simulink model "Bespiel_Architektur_Motor"  (R2025b)
settings: Solver=VariableStepAuto  StartTime=0.0  StopTime=1000  FixedStep=1  RelTol=1e-3
settings Model: DataDictionary=Bespiel_Architektur_Motor_dict.sldd  Creator=P28500  LastModifiedBy=P28500

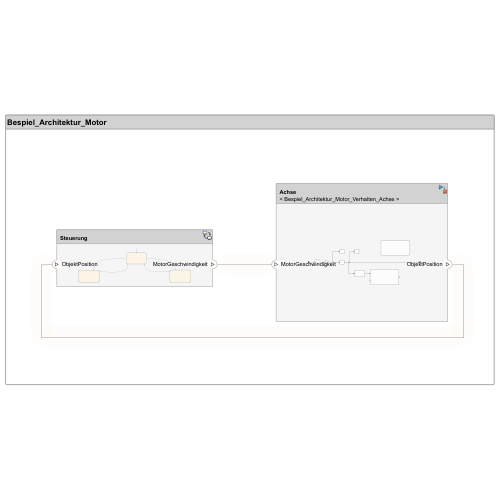
[thumbnail: Simulink's stored preview of the top-level diagram]
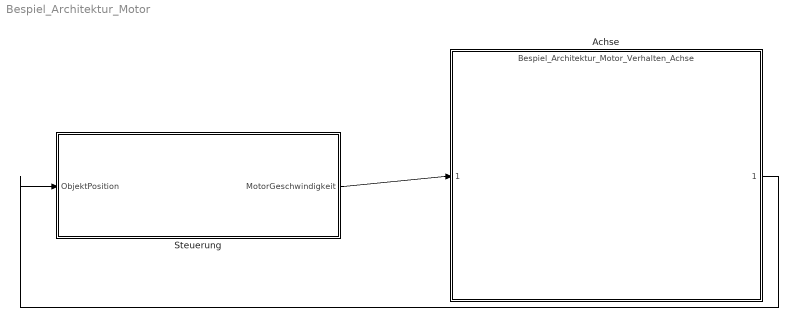
== system Bespiel_Architektur_Motor ==
  Achse : ModelReference  ModelNameDialog=Bespiel_Architektur_Motor_Verhalten_Achse  SimulationMode=Normal  ModelReferenceVersion=1.27
      settings: PortSchema="{\"entries\":[{\"content\":{\"headerSize\":38,\"margin\":15,\"minimumSpacing\":25,\"sides\":[{\"content\":{\"connectorIds\":[\"In1\"]},\"type\":\"ConnectorPlacement.EquallySpacedRectSide\",\"uuid\":\"9a345c98-45fd-4e3c-9541-4862f68f43a4\"},{\"content\":{\"connectorIds\":[\"Out1\"],\"side\":\"RIGHT\"},\"type\":\"ConnectorPlacement.EquallySpacedRectSide\",\"uuid\":\"9ac31d12-3781-423e-be76-ea02d94e9c74\"},{\"content\":{\"side\":\"TOP\"},\"type\":\"ConnectorPlacement.EquallySpacedRectSide\",\"uuid\":\"54d9933f-c35d-4577-9db1-9ffa0051924d\"}]},\"type\":\"ConnectorPlacement.EquallySpacedConnector\",\"uuid\":\"8ffce997-d126-4669-81c4-7f624f6ec4fc\"}],\"packageUris\":[\"http://schema.mathworks.com/mf0/Connector/R2020b\"],\"version\":\"1.0\"}"
  Steuerung : Stateflow chart  TreatAsAtomicUnit=on
      settings: PortSchema="{\"entries\":[{\"content\":{\"headerSize\":26,\"margin\":15,\"minimumSpacing\":25,\"sides\":[{\"content\":{\"connectorIds\":[\"In1\"]},\"type\":\"ConnectorPlacement.EquallySpacedRectSide\",\"uuid\":\"9a345c98-45fd-4e3c-9541-4862f68f43a4\"},{\"content\":{\"connectorIds\":[\"Out1\"],\"side\":\"RIGHT\"},\"type\":\"ConnectorPlacement.EquallySpacedRectSide\",\"uuid\":\"9ac31d12-3781-423e-be76-ea02d94e9c74\"},{\"content\":{\"side\":\"TOP\"},\"type\":\"ConnectorPlacement.EquallySpacedRectSide\",\"uuid\":\"54d9933f-c35d-4577-9db1-9ffa0051924d\"}]},\"type\":\"ConnectorPlacement.EquallySpacedConnector\",\"uuid\":\"8ffce997-d126-4669-81c4-7f624f6ec4fc\"}],\"packageUris\":[\"http://schema.mathworks.com/mf0/Connector/R2020b\"],\"version\":\"1.0\"}"
  wires:
  Steuerung/1(MotorGeschwindigkeit) -> Achse/1
  Achse/1 -> Steuerung/1(ObjektPosition)

== stateflow chart Bespiel_Architektur_Motor/Steuerung ==
  state Aus
    en:
    MotorGeschwindigkeit=0
    du:
    MotorGeschwindigkeit=0
  state Links_fahren
    en:
    MotorGeschwindigkeit=-0.1
    du:
    MotorGeschwindigkeit=-0.1
  state Rechts_fahren
    en:
    MotorGeschwindigkeit=0.1
    du:
    MotorGeschwindigkeit=0.1
  (default) -> Aus
  Aus -> Rechts_fahren [order 1] : [ObjektPosition<=0]{MotorGeschwindigkeit=0.1}
  Aus -> Links_fahren [order 2] : [ObjektPosition>=10]{MotorGeschwindigkeit=-0.1}
  Rechts_fahren -> Aus : [ObjektPosition>=10]{MotorGeschwindigkeit=0}
  Links_fahren -> Aus : [ObjektPosition<=0]{MotorGeschwindigkeit=0}
  data: ObjektPosition input double; MotorGeschwindigkeit output double
